simulink model "AFST_VD"  (R2016b)
settings: configuration reference "CodeGenConfigSet" (kept outside this file)
values from neighbouring files (symbols this model uses):
  Air_facPT1TAFS_C = Calibration.Parameter    [init_AFST_VD.m]    (also in init_AFST_VD_SIL.m = Simulink.Parameter)
  Air_RmpSlpTAFSNeg_C = Calibration.Parameter    [init_AFST_VD.m]    (also in init_AFST_VD_SIL.m = Simulink.Parameter)
  Air_RmpSlpTAFSPos_C = Calibration.Parameter    [init_AFST_VD.m]    (also in init_AFST_VD_SIL.m = Simulink.Parameter)
  Air_tTransStgTAFSDfl_C = Calibration.Parameter    [init_AFST_VD.m]    (also in init_AFST_VD_SIL.m = Simulink.Parameter)
  SigTst_swtTAFS_C = Calibration.Parameter    [init_AFST_VD.m]    (also in init_AFST_VD_SIL.m = Simulink.Parameter)
  SigTst_tTAFS_C = Calibration.Parameter    [init_AFST_VD.m]    (also in init_AFST_VD_SIL.m = Simulink.Parameter)
undefined symbols (not defined in the file or in its folder): AFST_VD_DT, Switch_conv
libraries: CXLib x4
settings Model: Creator=lenovo  LastModifiedBy=lenovo
settings ConfigSetRef: SourceLocation=Base Workspace

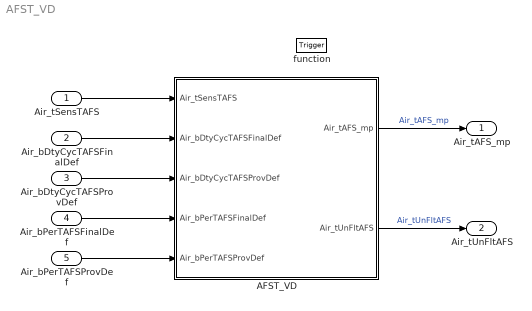
== system AFST_VD ==
  Air_tSensTAFS : Inport  Tag=deg  Description=Sensed value of the air temperature at HFM position  OutMin=-200  OutMax=200  OutDataTypeStr=Temp_deg
  Air_bDtyCycTAFSFinalDef : Inport  Description=Fault flag of TAFS Duty Cycle Final fault  Port=2  OutMin=0  OutMax=1  OutDataTypeStr=boolean
  Air_bDtyCycTAFSProvDef : Inport  Description=Fault flag of TAFS Duty Cycle fault Proving  Port=3  OutMin=0  OutMax=1  OutDataTypeStr=boolean
  Air_bPerTAFSFinalDef : Inport  Description=Fault flag of TAFS Period Final fault  Port=4  OutMin=0  OutMax=1  OutDataTypeStr=boolean
  Air_bPerTAFSProvDef : Inport  Description=Fault flag of TAFS Period fault Proving  Port=5  OutMin=0  OutMax=1  OutDataTypeStr=boolean
  function : TriggerPort  TriggerType=function-call  VariantControl=Variant
  AFST_VD : Subsystem
  Air_tAFS_mp : Outport  Tag=deg  Description=Induction air temperature at the HFM  OutMin=-200  OutMax=200  OutDataTypeStr=Temp_deg
  Air_tUnFltAFS : Outport  Tag=deg  Description=Charge-air temperature downstream from charge-air cooler  Port=2  OutMin=-200  OutMax=200  OutDataTypeStr=Temp_deg
  wires:
  AFST_VD/1(Air_tAFS_mp) -> Air_tAFS_mp/1  "Air_tAFS_mp"
  AFST_VD/2(Air_tUnFltAFS) -> Air_tUnFltAFS/1  "Air_tUnFltAFS"
  Air_tSensTAFS/1 -> AFST_VD/1(Air_tSensTAFS)
  Air_bDtyCycTAFSFinalDef/1 -> AFST_VD/2(Air_bDtyCycTAFSFinalDef)
  Air_bDtyCycTAFSProvDef/1 -> AFST_VD/3(Air_bDtyCycTAFSProvDef)
  Air_bPerTAFSFinalDef/1 -> AFST_VD/4(Air_bPerTAFSFinalDef)
  Air_bPerTAFSProvDef/1 -> AFST_VD/5(Air_bPerTAFSProvDef)

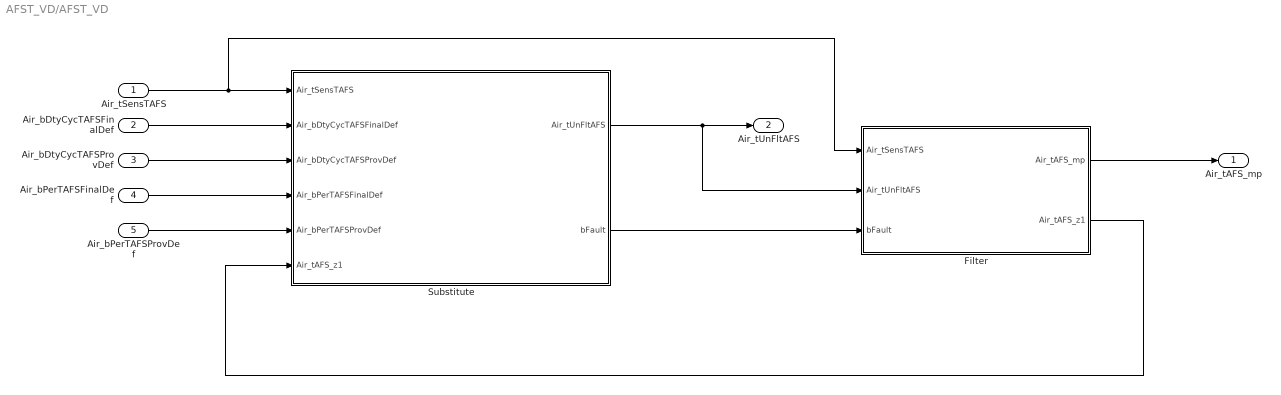
== system AFST_VD/AFST_VD ==
  Air_tSensTAFS : Inport  Tag=deg  Description=Sensed value of the air temperature at HFM position  OutMin=-200  OutMax=200  OutDataTypeStr=Temp_deg
  Air_bDtyCycTAFSFinalDef : Inport  Description=Fault flag of TAFS Duty Cycle Final fault  Port=2  OutMin=0  OutMax=1  OutDataTypeStr=boolean
  Air_bDtyCycTAFSProvDef : Inport  Description=Fault flag of TAFS Duty Cycle fault Proving  Port=3  OutMin=0  OutMax=1  OutDataTypeStr=boolean
  Air_bPerTAFSFinalDef : Inport  Description=Fault flag of TAFS Period Final fault  Port=4  OutMin=0  OutMax=1  OutDataTypeStr=boolean
  Air_bPerTAFSProvDef : Inport  Description=Fault flag of TAFS Period fault Proving  Port=5  OutMin=0  OutMax=1  OutDataTypeStr=boolean
  Filter : Subsystem
  Substitute : Subsystem
  Air_tAFS_mp : Outport  Tag=deg  Description=Induction air temperature at the HFM  OutMin=-200  OutMax=200  OutDataTypeStr=Temp_deg
  Air_tUnFltAFS : Outport  Tag=deg  Description=Charge-air temperature downstream from charge-air cooler  Port=2  OutMin=-200  OutMax=200  OutDataTypeStr=Temp_deg
  wires:
  Air_bDtyCycTAFSFinalDef/1 -> Substitute/2(Air_bDtyCycTAFSFinalDef)
  Air_bPerTAFSFinalDef/1 -> Substitute/4(Air_bPerTAFSFinalDef)
  Air_bDtyCycTAFSProvDef/1 -> Substitute/3(Air_bDtyCycTAFSProvDef)
  Air_bPerTAFSProvDef/1 -> Substitute/5(Air_bPerTAFSProvDef)
  Air_tSensTAFS/1 -> Substitute/1(Air_tSensTAFS), Filter/1(Air_tSensTAFS)
  Substitute/1(Air_tUnFltAFS) -> Filter/2(Air_tUnFltAFS), Air_tUnFltAFS/1
  Filter/1(Air_tAFS_mp) -> Air_tAFS_mp/1
  Filter/2(Air_tAFS_z1) -> Substitute/6(Air_tAFS_z1)
  Substitute/2(bFault) -> Filter/3(bFault)

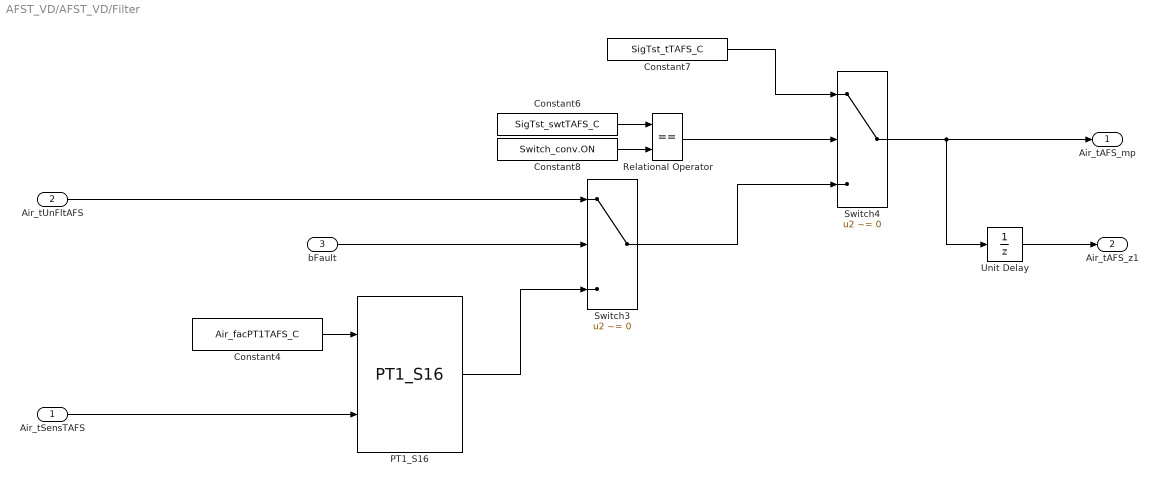
== system AFST_VD/AFST_VD/Filter ==
  Air_tSensTAFS : Inport
  Air_tUnFltAFS : Inport  Port=2
  bFault : Inport  Port=3
  Constant4 : Constant  Value=Air_facPT1TAFS_C
  Constant6 : Constant  Value=SigTst_swtTAFS_C
  Constant7 : Constant  Value=SigTst_tTAFS_C
  Constant8 : Constant  Value=Switch_conv.ON
  PT1_S16 : CXLib/PT1_S16  offset=2731.4
  Relational Operator : RelationalOperator  Operator===  OutDataTypeStr=boolean  RndMeth=Simplest
  Switch3 : Switch  Criteria=u2 ~= 0
  Switch4 : Switch  Criteria=u2 ~= 0
  Unit Delay : UnitDelay  SampleTime=-1
      settings: AttributesFormatString=InitialValue=%<InitialCondition>
  Air_tAFS_mp : Outport
  Air_tAFS_z1 : Outport  Port=2
  wires:
  Switch3/1 -> Switch4/3
  Constant6/1 -> Relational Operator/1
  Constant8/1 -> Relational Operator/2
  Relational Operator/1 -> Switch4/2
  Constant7/1 -> Switch4/1
  Switch4/1 -> Unit Delay/1, Air_tAFS_mp/1
  Air_tUnFltAFS/1 -> Switch3/1
  Constant4/1 -> PT1_S16/1
  Unit Delay/1 -> Air_tAFS_z1/1
  bFault/1 -> Switch3/2
  PT1_S16/1 -> Switch3/3
  Air_tSensTAFS/1 -> PT1_S16/2

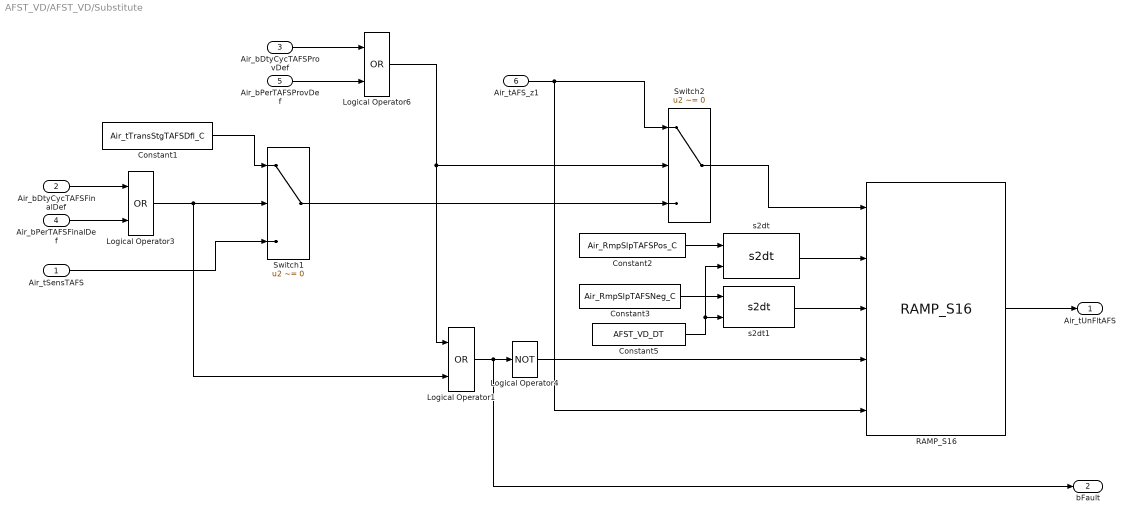
== system AFST_VD/AFST_VD/Substitute ==
  Air_tSensTAFS : Inport
  Air_bDtyCycTAFSFinalDef : Inport  Port=2
  Air_bDtyCycTAFSProvDef : Inport  Description=Fault flag of TAFS Duty Cycle fault Proving  Port=3  OutMin=0  OutMax=1  OutDataTypeStr=boolean
  Air_bPerTAFSFinalDef : Inport  Port=4
  Air_bPerTAFSProvDef : Inport  Description=Fault flag of TAFS Period fault Proving  Port=5  OutMin=0  OutMax=1  OutDataTypeStr=boolean
  Air_tAFS_z1 : Inport  Port=6
  Constant1 : Constant  Value=Air_tTransStgTAFSDfl_C
  Constant2 : Constant  Value=Air_RmpSlpTAFSPos_C
  Constant3 : Constant  Value=Air_RmpSlpTAFSNeg_C
  Constant5 : Constant  Value=AFST_VD_DT
  Logical Operator1 : Logic  Operator=OR  AllPortsSameDT=off  OutDataTypeStr=boolean
  Logical Operator3 : Logic  Operator=OR  AllPortsSameDT=off  OutDataTypeStr=boolean
  Logical Operator4 : Logic  Operator=NOT  AllPortsSameDT=off  OutDataTypeStr=boolean
  Logical Operator6 : Logic  Operator=OR  AllPortsSameDT=off  OutDataTypeStr=boolean
  RAMP_S16 : CXLib/RAMP_S16
  Switch1 : Switch  Criteria=u2 ~= 0
  Switch2 : Switch  Criteria=u2 ~= 0
  s2dt : CXLib/s2dt
  s2dt1 : CXLib/s2dt
  Air_tUnFltAFS : Outport
  bFault : Outport  Port=2
  wires:
  Air_tSensTAFS/1 -> Switch1/3
  s2dt/1 -> RAMP_S16/2
  s2dt1/1 -> RAMP_S16/3
  Constant2/1 -> s2dt/1
  Constant3/1 -> s2dt1/1
  Constant5/1 -> s2dt/2, s2dt1/2
  Air_bDtyCycTAFSFinalDef/1 -> Logical Operator3/1
  Air_bPerTAFSFinalDef/1 -> Logical Operator3/2
  Logical Operator4/1 -> RAMP_S16/4
  Logical Operator3/1 -> Logical Operator1/2, Switch1/2
  Air_bPerTAFSProvDef/1 -> Logical Operator6/2
  Air_bDtyCycTAFSProvDef/1 -> Logical Operator6/1
  Logical Operator6/1 -> Switch2/2, Logical Operator1/1
  Air_tAFS_z1/1 -> RAMP_S16/5, Switch2/1
  Switch1/1 -> Switch2/3
  Constant1/1 -> Switch1/1
  Switch2/1 -> RAMP_S16/1
  RAMP_S16/1 -> Air_tUnFltAFS/1
  Logical Operator1/1 -> bFault/1, Logical Operator4/1
